simulink model "BatterySOCSimulinkEstimation"  (R2023a)
settings: Solver=VariableStepAuto  StartTime=0.0  StopTime=timeVector(end)  RelTol=1e-3
values from neighbouring files (symbols this model uses):
  X_MAX = [4.23207255751 5.99961 26.28963]    [BatteryData.mat]
  X_MIN = [2.79645479834 -18.0971537397 -10.3047309401]    [BatteryData.mat]
libraries: deeplib x1
settings Model: Creator=The MathWorks, Inc.  LastModifiedBy=The MathWorks, Inc.
settings SolverCC: MaxZcPerStep=1
settings DebuggingCC: UnconnectedInputMsg=warning  UnconnectedOutputMsg=warning  UnconnectedLineMsg=warning
settings ModelReferenceCC: EnableRefExpFcnMdlSchedulingChecks=on
settings RTWCC: DLArmComputeVersion=19.05

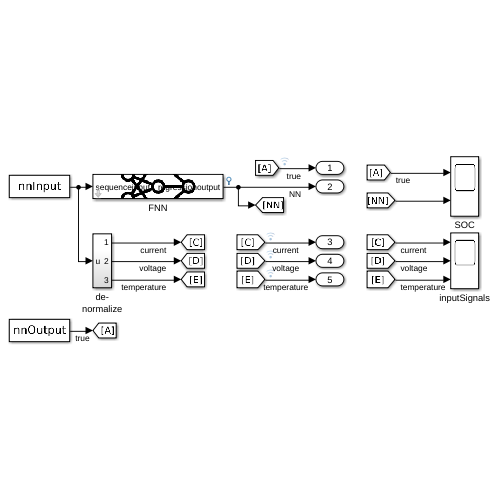
[thumbnail: Simulink's stored preview of the top-level diagram]
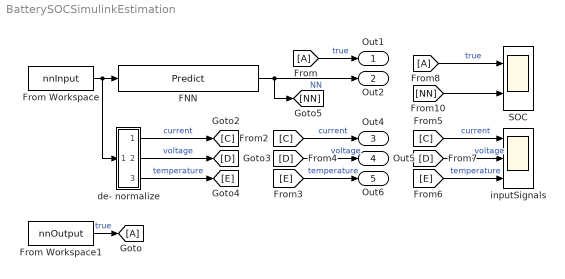
== system BatterySOCSimulinkEstimation ==
  FNN : deeplib/Predict  Network=Network from MAT-file  NetworkFunction=squeezenet  NetworkFilePath=battery_SOC_net.mat  MiniBatchSize=1  InputDataFormats={ '', '' }  Predictions=on  Activations={}  ForceInterpretedSim=off  EnableDLNetwork=off
  From : From
  From Workspace : FromWorkspace  VariableName=nnInput
  From Workspace1 : FromWorkspace  VariableName=nnOutput
  From8 : From
  Goto : Goto
  SOC : Scope  NumInputPorts=2
  de- normalize : Subsystem
  inputSignals : Scope  NumInputPorts=3
  Out1 : Outport
  Out2 : Outport  Port=2
  Out4 : Outport  Port=3
  Out5 : Outport  Port=4
  Out6 : Outport  Port=5
  wires:
  [NN] -> SOC/2
  [E] -> Out6/1  "temperature"
  From/1 -> Out1/1  "true"
  [E] -> inputSignals/3  "temperature"
  From8/1 -> SOC/1  "true"
  [D] -> Out5/1  "voltage"
  de- normalize/3(Out3) -> [E]  "temperature"
  [C] -> inputSignals/1  "current"
  [D] -> inputSignals/2  "voltage"
  de- normalize/2(Out2) -> [D]  "voltage"
  From Workspace/1 -> FNN/1, de- normalize/1(u)
  [C] -> Out4/1  "current"
  FNN/1 -> [NN], Out2/1  "NN"
  de- normalize/1(Out1) -> [C]  "current"
  From Workspace1/1 -> Goto/1  "true"

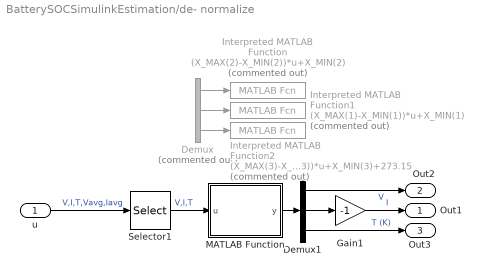
== system BatterySOCSimulinkEstimation/de- normalize ==
  u : Inport
  Demux : Demux  Commented=on  Outputs=3
  Demux1 : Demux  Outputs=3
  Gain1 : Gain  Gain=-1
  Interpreted MATLAB Function : MATLABFcn  Commented=on  MATLABFcn=(X_MAX(2)-X_MIN(2))*u+X_MIN(2)
  Interpreted MATLAB Function1 : MATLABFcn  Commented=on  MATLABFcn=(X_MAX(1)-X_MIN(1))*u+X_MIN(1)
  Interpreted MATLAB Function2 : MATLABFcn  Commented=on  MATLABFcn=(X_MAX(3)-X_MIN(3))*u+X_MIN(3)+273.15
  MATLAB Function : MATLAB Function  TreatAsAtomicUnit=on
  Selector1 : Selector  InputPortWidth=5  IndexOptions=Index vector (dialog)  Indices=[1 2 3]  OutputSizes=1
  Out1 : Outport
  Out2 : Outport  Port=2
  Out3 : Outport  Port=3
  wires:
  Demux/3 -> Interpreted MATLAB Function2/1
  Demux/1 -> Interpreted MATLAB Function/1
  u/1 -> Selector1/1  "V,I,T,Vavg,Iavg"
  Demux/2 -> Interpreted MATLAB Function1/1
  MATLAB Function/1(y) -> Demux1/1
  Demux1/3 -> Out3/1  "T (K)"
  Demux1/1 -> Out2/1  "V"
  Demux1/2 -> Gain1/1
  Selector1/1 -> MATLAB Function/1(u)  "V,I,T"
  Gain1/1 -> Out1/1  "I"

== matlab function BatterySOCSimulinkEstimation/de- normalize/MATLAB Function ==
  data: u input; y output; X_MAX parameter; X_MIN parameter
function y = fcn(u, X_MAX, X_MIN)
y = (X_MAX-X_MIN).*u+X_MIN;
y(3) = y(3) + 273.15; % convert to K
